simulink model "AC2DC_Converter"  (R2019a)
settings: Solver=ode23t  StartTime=0.0  StopTime=0.5  FixedStep=Ts  MaxStep=1e-4  RelTol=1e-3  EnableMultiTasking=on
PreLoadFcn:
  | pe_buck_converter_control_data;
undefined symbols (not defined in the file): RL, Ts, Tsc, Vref
libraries: fl_lib x12, nesl_utility x6, ee_lib x5, eeDcDcVoltageController x1, eePwmGenerator x1, dspstat3 x1
CloseFcn:
  | try,close(h1_pe_buck_converter_control),end
  | clear h1_pe_buck_converter_control
  | 
  | clear simlog_pe_buck_converter_control
  | clear logsout_pe_buck_converter_control
Description:
  | Buck Converter Voltage Control
  | 
  | Copyright 2017 The MathWorks, Inc.
settings Model: Creator=The MathWorks, Inc.  LastModifiedBy=jcale
settings DataIOCC: MaxDataPoints=210000  ReturnWorkspaceOutputs=off  SignalLoggingName=logsout_pe_buck_converter_control
settings OptimizationCC: LifeSpan=inf
settings DebuggingCC: UnderspecifiedInitializationDetection=Classic  MergeDetectMultiDrivingBlocksExec=none  PregeneratedLibrarySubsystemCodeDiagnostic=none  SFUnexpectedBacktrackingDiag=warning  SFNoUnconditionalDefaultTransitionDiag=warning  SFExecutionAtInitializationDiag=none  ArithmeticOperatorsInVariantConditions=warning
settings SFSimCC: SimUseLocalCustomCode=off
settings RTWCC: RTWUseLocalCustomCode=off
settings CodeAppCC: StateflowObjectComments=on
settings GRTTargetCC: TargetLangStandard=C89/C90 (ANSI)  GeneratePreprocessorConditionals=Disable all
settings ConfigComp: CovMetricSettings=dw  CovHtmlReporting=on  CovSaveCumulativeToWorkspaceVar=on  CovSaveSingleToWorkspaceVar=on  CovExternalEMLEnable=off
settings SimscapeCC: SimscapeNormalizeSystem=off  SimscapeLogType=all  SimscapeLogSimulationStatistics=on  SimscapeLogName=simlog_pe_buck_converter_control  SimscapeLogDataHistory=210000

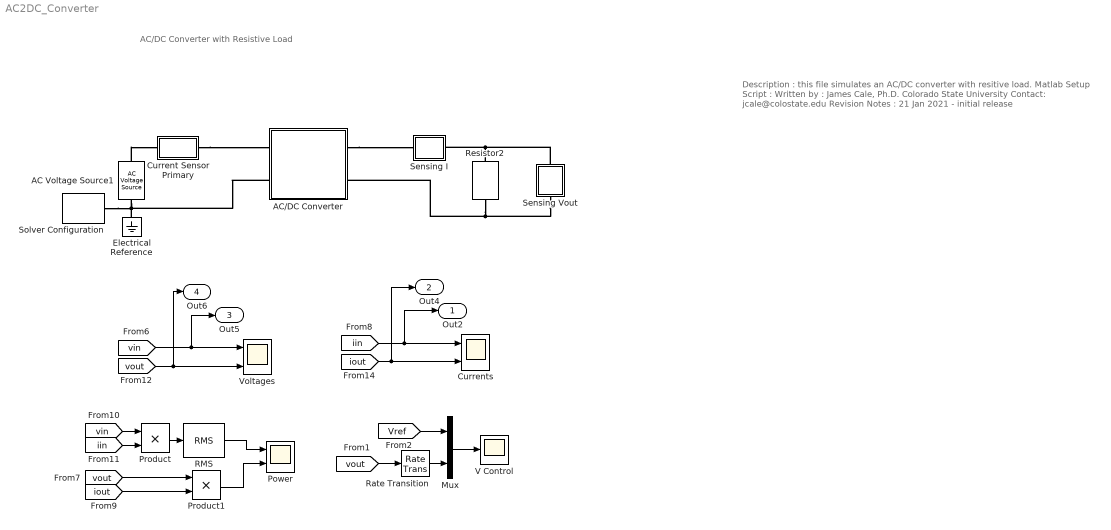
== system AC2DC_Converter ==
  note: AC/DC Converter with Resistive Load
  note: Description : this file simulates an AC/DC converter with resitive load.
      |
      | Matlab Setup Script :
      |
      | Written by :
      | James Cale, Ph.D.
      | Colorado State University
      | Contact: jcale@colostate.edu
      |
      | Revision Notes :
      | 21 Jan 2021 - initial release
  AC Voltage Source1 : fl_lib/Electrical/Electrical Sources/AC Voltage Source  amp=178 V  shift=-90 deg  frequency=60 Hz  omega=0 rad/s
  AC/DC Converter : Subsystem  mask{r_line=5e-1, l_line=1e-4, c_f=100e-6, r_f=5e-1, Kp=0.0547, Ki=8.8644}
      mask prompts: r_line "Input line resistance (Ohm)"; l_line "Input line inductance (H)"; c_f "Input filter capacitor (F)"; r_f "Input filter resistor (Ohm)"; Kp "Controller proportional gain"; Ki "Controller integrator gain"
      mask Display:
      | %disp('AC/DC Converter')
      | %pos = get_param(gcb,'Position')
      | %plot([pos(1) pos(2)],[pos(3) pos(4)])
      | plot([0.25 0.75], [.25 .25])
      | plot([0.75 0.75], [.25 0.75])
      | plot([0.75 0.25], [0.75 0.75])
      | plot([0.25 0.25], [0.75 .25])
      | plot([0.25 0.25], [0.75 .25])
      | 
      | plot([0.25 0.75], [0.25 .75])
      | 
      | text(.35,.62, '{\fontsize{20}~}','texmode','on')
      | text(.6,.45, '{\fontsize{20}-}','texmode','on')
  Current Sensor Primary : Subsystem
      mask Display: disp('v, i', 'texmode','on')
  Currents : Scope  NumInputPorts=2
  Electrical Reference : fl_lib/Electrical/Electrical Elements/Electrical Reference
  Mux : Mux  Inputs=2
  Power : Scope  NumInputPorts=2
  Product : Product
  Product1 : Product
  RMS : dspstat3/RMS  run=on  directionMode=Each column  dimension=1  InputProcessing=Columns as channels (frame based)  reset_popup=None
  Rate Transition : RateTransition  OutPortSampleTime=Tsc
  Resistor2 : fl_lib/Electrical/Electrical Elements/Resistor  R=RL Ohm  i_specify=off  i_priority=None  i=0 A  i_nominal_specify=off  i_nominal_unit=A  i_nominal_value=1  v_specify=off  v_priority=None  v=0 V  v_nominal_specify=off  v_nominal_unit=V  v_nominal_value=1
  Sensing Vout : Subsystem
      mask Display:
      | disp('v')
      | %port_label('Lconn',1,'+')
      | %port_label('Rconn',1,'-')
  Sensing I : Subsystem
      mask Display:
      | disp('i')
      | %port_label('Lconn',1,'+')
      | %port_label('Rconn',1,'-')
  Solver Configuration : nesl_utility/Solver Configuration  PhysicalDomain=network_engine_domain  SubClassName=solver  LeftPortType=input  RightPortType=generic  Tones=[]  Harmonics=[]  SimulateNoise=off  Profile=off  UseLocalSampling=off  EnableSwitchedLinearOptims=on  FrequencyDomain=off  UseCCode=off  RelTol=0.001  AbsTol=1e-06  MinStep=1e-09  ToWorkspace=off  RevertToSquareIcSolve=off  NumHomotopyIterations=100  PhasorMode=off  PhasorModeNumHarmonics=1  DoDC=off  ResidualTolerance=1e-9  UseLocalSolver=on  LocalSolverChoice=NE_BACKWARD_EULER_ADVANCER  LocalSolverSampleTime=Ts  DoFixedCost=on  MaxNonlinIter=3  MaxModeIter=2  LinearAlgebra=auto  EquationFormulation=NE_TIME_EF  DelaysMemoryBudget=1024  AutomaticFiltering=on  FilteringTimeConstant=0.001  PartitionStorageMethod=AS_NEEDED  PartitionMemoryBudget=1024  PartitionMethod=FAST
  V Control : Scope
  Voltages : Scope  NumInputPorts=2
  Out2 : Outport  SignalName=iin  InitialOutput=0
  Out4 : Outport  Port=2  SignalName=iout  InitialOutput=0
  Out5 : Outport  Port=3  SignalName=vin  InitialOutput=0
  Out6 : Outport  Port=4  SignalName=vout  InitialOutput=0
  wires:
  [vout] -> Rate Transition/1
  Mux/1 -> V Control/1
  [Vref] -> Mux/1
  Rate Transition/1 -> Mux/2
  Product/1 -> RMS/1
  [vout] -> Voltages/2, Out6/1
  [iin] -> Currents/1, Out2/1
  [iout] -> Currents/2, Out4/1
  [vin] -> Voltages/1, Out5/1
  RMS/1 -> Power/1
  [vout] -> Product1/1
  [iout] -> Product1/2
  [vin] -> Product/1
  [iin] -> Product/2
  Product1/1 -> Power/2
  connections:
  Resistor2/RConn1 -- AC/DC Converter/RConn2 -- Sensing Vout/RConn1
  Electrical Reference/LConn1 -- Solver Configuration/RConn1 -- AC/DC Converter/LConn2 -- AC Voltage Source1/RConn1
  AC Voltage Source1/LConn1 -- Current Sensor Primary/LConn1
  Current Sensor Primary/RConn1 -- AC/DC Converter/LConn1
  AC/DC Converter/RConn1 -- Sensing I/LConn1
  Sensing Vout/LConn1 -- Resistor2/LConn1 -- Sensing I/RConn1

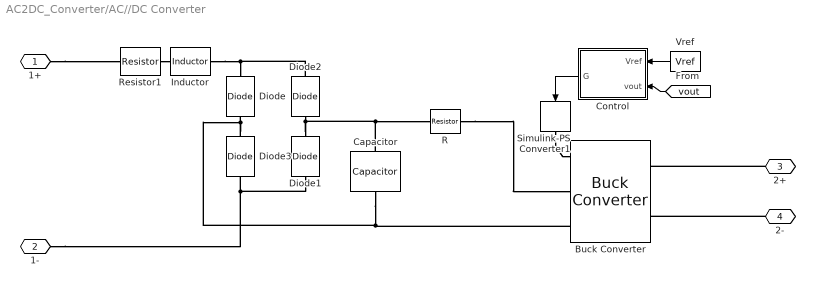
== system AC2DC_Converter/AC//DC Converter ==
  Buck Converter : ee_lib/Semiconductors & Converters/Converters/Buck Converter  device_type=3  Vf=0.8 V  Ron=0.001 Ohm  Rds=0.001 Ohm  Goff=1e-5 1/Ohm  Vth=0.5 V  Vgt=1 V  Vgt_off=-1 V  Ih=1 A  diode_param=2  diode_Vf=0.8 V  diode_Ron=0.001 Ohm  diode_Goff=1e-5 1/Ohm  diode_C=50 nF  diode_iRM=-235 A  diode_iF=300 A  diode_idot=-50 A/us  diode_trr_param=1  diode_trr_factor=3  diode_trr=15 us  diode_Qrr=1500 s*uA  Lf=3.7e-2 H  Cf=1e-5 F  Rf=0.01 Ohm  snubber_type=0  Rs=0.1 Ohm  Cs=1e-7 F
      settings: SourceProductName=Simscape Electrical  SourceProductBaseCode=PS
  Capacitor : fl_lib/Electrical/Electrical Elements/Capacitor  c=c_f F  r=1e-6 Ohm  g=0 1/Ohm  i_specify=off  i_priority=None  i=0 A  i_nominal_specify=off  i_nominal_unit=A  i_nominal_value=1  v_specify=off  v_priority=None  v=0 V  v_nominal_specify=off  v_nominal_unit=V  v_nominal_value=1  vc_specify=off  vc_priority=High  vc=0 V  vc_nominal_specify=off  vc_nominal_unit=V  vc_nominal_value=1
  Control : Subsystem
  Diode : ee_lib/Semiconductors & Converters/Diode  ModelType=ee.enum.diode.modelType.pwl  Vf=.5 V  Ron=0.2 Ohm  Goff=1e-8 S  prmExp=1  I12=[.0137, .545] A  V12=[.6, .7] V  IS=1e-12 A  ec=1  I1=0.0137 A  V1=0.6 V  RS=0.01 Ohm  Tmeas=25 degC  N_series=1  N_parallel=1  Rz=0.3 Ohm  BV=inf V  C_param=1  CJ=5 pF  CJ0=5 pF  VJ=1 V  Mgrad=0.5  Vvec=[.1, 10, 100] V  Cvec=[3.5, 1, .4] pF  FC=0.5  Q_param=ee.enum.diode.recoveryParam.off  iRM=-7.15 A  iF=4 A  didt=-750 A/us  trr_factor=3  trr=115 ns  Qrr=1500 s*uA  TT=50 ns  tau=100 ns  T_param=1  IS_T2=1.25e-7 A  I1_T2=0.245 A  V1_T2=0.5 V  Tmeas2=125 degC  EG_param=1  EG=1.11 eV  XTI_param=1  XTI=3  dBVdT=0 V/K  Tdevice=25 degC  i_specify=off  i_priority=None  i=0 A  i_nominal_specify=off  i_nominal_unit=A  i_nominal_value=1  v_specify=off  v_priority=None  v=0 V  v_nominal_specify=off  v_nominal_unit=V  v_nominal_value=1  i_capacitor_specify=off  i_capacitor_priority=High  i_capacitor=0 A  i_capacitor_nominal_specify=off  i_capacitor_nominal_unit=A  i_capacitor_nominal_value=1  v_capacitor_specify=off  v_capacitor_priority=None  v_capacitor=0 V  v_capacitor_nominal_specify=off  v_capacitor_nominal_unit=V  v_capacitor_nominal_value=1  power_dissipated_specify=off  power_dissipated_priority=None  power_dissipated=0 W  power_dissipated_nominal_specify=off  power_dissipated_nominal_unit=W  power_dissipated_nominal_value=1  Rth=[0, 10] K/W  thermal_mass_parameterization=ee.enum.thermalNetwork.timeconstant  thermal_mass=[0, 1] J/K  thermal_time_constant=[0, 10] s  thermal_mass_initial_temperatures=[25, 25] degC
      settings: SourceProductName=Simscape Electrical
  Diode1 : ee_lib/Semiconductors & Converters/Diode  ModelType=ee.enum.diode.modelType.pwl  Vf=.5 mV  Ron=0.2 Ohm  Goff=1e-8 S  prmExp=1  I12=[.0137, .545] A  V12=[.6, .7] V  IS=1e-12 A  ec=1  I1=0.0137 A  V1=0.6 V  RS=0.01 Ohm  Tmeas=25 degC  N_series=1  N_parallel=1  Rz=0.3 Ohm  BV=inf V  C_param=1  CJ=5 pF  CJ0=5 pF  VJ=1 V  Mgrad=0.5  Vvec=[.1, 10, 100] V  Cvec=[3.5, 1, .4] pF  FC=0.5  Q_param=ee.enum.diode.recoveryParam.off  iRM=-7.15 A  iF=4 A  didt=-750 A/us  trr_factor=3  trr=115 ns  Qrr=1500 s*uA  TT=50 ns  tau=100 ns  T_param=1  IS_T2=1.25e-7 A  I1_T2=0.245 A  V1_T2=0.5 V  Tmeas2=125 degC  EG_param=1  EG=1.11 eV  XTI_param=1  XTI=3  dBVdT=0 V/K  Tdevice=25 degC  i_specify=off  i_priority=None  i=0 A  i_nominal_specify=off  i_nominal_unit=A  i_nominal_value=1  v_specify=off  v_priority=None  v=0 V  v_nominal_specify=off  v_nominal_unit=V  v_nominal_value=1  i_capacitor_specify=off  i_capacitor_priority=High  i_capacitor=0 A  i_capacitor_nominal_specify=off  i_capacitor_nominal_unit=A  i_capacitor_nominal_value=1  v_capacitor_specify=off  v_capacitor_priority=None  v_capacitor=0 V  v_capacitor_nominal_specify=off  v_capacitor_nominal_unit=V  v_capacitor_nominal_value=1  power_dissipated_specify=off  power_dissipated_priority=None  power_dissipated=0 W  power_dissipated_nominal_specify=off  power_dissipated_nominal_unit=W  power_dissipated_nominal_value=1  Rth=[0, 10] K/W  thermal_mass_parameterization=ee.enum.thermalNetwork.timeconstant  thermal_mass=[0, 1] J/K  thermal_time_constant=[0, 10] s  thermal_mass_initial_temperatures=[25, 25] degC
      settings: SourceProductName=Simscape Electrical
  Diode2 : ee_lib/Semiconductors & Converters/Diode  ModelType=ee.enum.diode.modelType.pwl  Vf=.5 V  Ron=0.2 Ohm  Goff=1e-8 S  prmExp=1  I12=[.0137, .545] A  V12=[.6, .7] V  IS=1e-12 A  ec=1  I1=0.0137 A  V1=0.6 V  RS=0.01 Ohm  Tmeas=25 degC  N_series=1  N_parallel=1  Rz=0.3 Ohm  BV=inf V  C_param=1  CJ=5 pF  CJ0=5 pF  VJ=1 V  Mgrad=0.5  Vvec=[.1, 10, 100] V  Cvec=[3.5, 1, .4] pF  FC=0.5  Q_param=ee.enum.diode.recoveryParam.off  iRM=-7.15 A  iF=4 A  didt=-750 A/us  trr_factor=3  trr=115 ns  Qrr=1500 s*uA  TT=50 ns  tau=100 ns  T_param=1  IS_T2=1.25e-7 A  I1_T2=0.245 A  V1_T2=0.5 V  Tmeas2=125 degC  EG_param=1  EG=1.11 eV  XTI_param=1  XTI=3  dBVdT=0 V/K  Tdevice=25 degC  i_specify=off  i_priority=None  i=0 A  i_nominal_specify=off  i_nominal_unit=A  i_nominal_value=1  v_specify=off  v_priority=None  v=0 V  v_nominal_specify=off  v_nominal_unit=V  v_nominal_value=1  i_capacitor_specify=off  i_capacitor_priority=High  i_capacitor=0 A  i_capacitor_nominal_specify=off  i_capacitor_nominal_unit=A  i_capacitor_nominal_value=1  v_capacitor_specify=off  v_capacitor_priority=None  v_capacitor=0 V  v_capacitor_nominal_specify=off  v_capacitor_nominal_unit=V  v_capacitor_nominal_value=1  power_dissipated_specify=off  power_dissipated_priority=None  power_dissipated=0 W  power_dissipated_nominal_specify=off  power_dissipated_nominal_unit=W  power_dissipated_nominal_value=1  Rth=[0, 10] K/W  thermal_mass_parameterization=ee.enum.thermalNetwork.timeconstant  thermal_mass=[0, 1] J/K  thermal_time_constant=[0, 10] s  thermal_mass_initial_temperatures=[25, 25] degC
      settings: SourceProductName=Simscape Electrical
  Diode3 : ee_lib/Semiconductors & Converters/Diode  ModelType=ee.enum.diode.modelType.pwl  Vf=.5 V  Ron=0.2 Ohm  Goff=1e-8 S  prmExp=1  I12=[.0137, .545] A  V12=[.6, .7] V  IS=1e-12 A  ec=1  I1=0.0137 A  V1=0.6 V  RS=0.01 Ohm  Tmeas=25 degC  N_series=1  N_parallel=1  Rz=0.3 Ohm  BV=inf V  C_param=1  CJ=5 pF  CJ0=5 pF  VJ=1 V  Mgrad=0.5  Vvec=[.1, 10, 100] V  Cvec=[3.5, 1, .4] pF  FC=0.5  Q_param=ee.enum.diode.recoveryParam.off  iRM=-7.15 A  iF=4 A  didt=-750 A/us  trr_factor=3  trr=115 ns  Qrr=1500 s*uA  TT=50 ns  tau=100 ns  T_param=1  IS_T2=1.25e-7 A  I1_T2=0.245 A  V1_T2=0.5 V  Tmeas2=125 degC  EG_param=1  EG=1.11 eV  XTI_param=1  XTI=3  dBVdT=0 V/K  Tdevice=25 degC  i_specify=off  i_priority=None  i=0 A  i_nominal_specify=off  i_nominal_unit=A  i_nominal_value=1  v_specify=off  v_priority=None  v=0 V  v_nominal_specify=off  v_nominal_unit=V  v_nominal_value=1  i_capacitor_specify=off  i_capacitor_priority=High  i_capacitor=0 A  i_capacitor_nominal_specify=off  i_capacitor_nominal_unit=A  i_capacitor_nominal_value=1  v_capacitor_specify=off  v_capacitor_priority=None  v_capacitor=0 V  v_capacitor_nominal_specify=off  v_capacitor_nominal_unit=V  v_capacitor_nominal_value=1  power_dissipated_specify=off  power_dissipated_priority=None  power_dissipated=0 W  power_dissipated_nominal_specify=off  power_dissipated_nominal_unit=W  power_dissipated_nominal_value=1  Rth=[0, 10] K/W  thermal_mass_parameterization=ee.enum.thermalNetwork.timeconstant  thermal_mass=[0, 1] J/K  thermal_time_constant=[0, 10] s  thermal_mass_initial_temperatures=[25, 25] degC
      settings: SourceProductName=Simscape Electrical
  Inductor : fl_lib/Electrical/Electrical Elements/Inductor  l=l_line H  r=0 Ohm  g=1e-9 1/Ohm  i_specify=off  i_priority=None  i=0 A  i_nominal_specify=off  i_nominal_unit=A  i_nominal_value=1  v_specify=off  v_priority=None  v=0 V  v_nominal_specify=off  v_nominal_unit=V  v_nominal_value=1  i_L_specify=off  i_L_priority=High  i_L=0 A  i_L_nominal_specify=off  i_L_nominal_unit=A  i_L_nominal_value=1
  R : fl_lib/Electrical/Electrical Elements/Resistor  R=r_f Ohm  i_specify=off  i_priority=None  i=0 A  i_nominal_specify=off  i_nominal_unit=A  i_nominal_value=1  v_specify=off  v_priority=None  v=0 V  v_nominal_specify=off  v_nominal_unit=V  v_nominal_value=1
      settings: SourceProductName=Foundation Library
  Resistor1 : fl_lib/Electrical/Electrical Elements/Resistor  R=r_line Ohm  i_specify=off  i_priority=None  i=0 A  i_nominal_specify=off  i_nominal_unit=A  i_nominal_value=1  v_specify=off  v_priority=None  v=0 V  v_nominal_specify=off  v_nominal_unit=V  v_nominal_value=1
  Simulink-PS Converter1 : nesl_utility/Simulink-PS Converter  PhysicalDomain=network_engine_domain  SubClassName=ps_input  LeftPortType=input  RightPortType=output  PseudoPeriodic=off  Frequencies=[]  NoiseDistribution=none  NoiseParameters=[]  Unit=1  AffineConversion=off  FilteringAndDerivatives=provide  SimscapeFilterOrder=1  InputFilterTimeConstant=0.001  UdotUserProvided=0
  Vref : Constant  Value=Vref  SampleTime=Ts
  1+ : PMIOPort  Side=Left
  1- : PMIOPort  Port=2  Side=Left
  2+ : PMIOPort  Port=3  Side=Right
  2- : PMIOPort  Port=4  Side=Right
  wires:
  [vout] -> Control/2(vout)
  Control/1(G) -> Simulink-PS Converter1/1
  Vref/1 -> Control/1(Vref)
  connections:
  2-/RConn1 -- Buck Converter/RConn2
  1+/RConn1 -- Resistor1/LConn1
  2+/RConn1 -- Buck Converter/RConn1
  Simulink-PS Converter1/RConn1 -- Buck Converter/LConn1
  Diode3/RConn1 -- 1-/RConn1 -- Diode1/LConn1
  Resistor1/RConn1 -- Inductor/LConn1
  R/RConn1 -- Buck Converter/LConn2
  Diode/RConn1 -- Diode2/LConn1 -- Inductor/RConn1
  Diode/LConn1 -- Capacitor/RConn1 -- Buck Converter/LConn3 -- Diode3/LConn1
  Capacitor/LConn1 -- Diode2/RConn1 -- Diode1/RConn1 -- R/LConn1

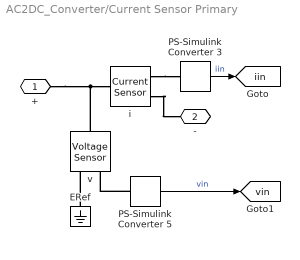
== system AC2DC_Converter/Current Sensor Primary ==
  ERef : fl_lib/Electrical/Electrical Elements/Electrical Reference
  PS-Simulink Converter 3 : nesl_utility/PS-Simulink Converter  PhysicalDomain=network_engine_domain  SubClassName=ps_output  LeftPortType=input  RightPortType=output  PseudoPeriodic=off  Frequencies=[]  Unit=1  AffineConversion=off
  PS-Simulink Converter 5 : nesl_utility/PS-Simulink Converter  PhysicalDomain=network_engine_domain  SubClassName=ps_output  LeftPortType=input  RightPortType=output  PseudoPeriodic=off  Frequencies=[]  Unit=1  AffineConversion=off
  i : fl_lib/Electrical/Electrical Sensors/Current Sensor
  v : fl_lib/Electrical/Electrical Sensors/Voltage Sensor
  + : PMIOPort  Side=Left
  - : PMIOPort  Port=2  Side=Right
  tag scope: iin=global, vin=global
  wires:
  PS-Simulink Converter 3/1 -> [iin]  "iin"
  PS-Simulink Converter 5/1 -> [vin]  "vin"
  connections:
  i/RConn2 -- -/RConn1
  +/RConn1 -- v/LConn1 -- i/LConn1
  i/RConn1 -- PS-Simulink Converter 3/LConn1
  PS-Simulink Converter 5/LConn1 -- v/RConn1
  ERef/LConn1 -- v/RConn2

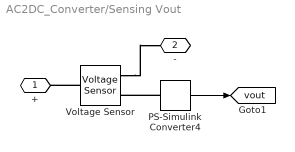
== system AC2DC_Converter/Sensing Vout ==
  PS-Simulink Converter4 : nesl_utility/PS-Simulink Converter  PhysicalDomain=network_engine_domain  SubClassName=ps_output  LeftPortType=input  RightPortType=output  PseudoPeriodic=off  Frequencies=[]  Unit=V  AffineConversion=off
  Voltage Sensor : fl_lib/Electrical/Electrical Sensors/Voltage Sensor
      settings: SourceProductName=Foundation Library
  + : PMIOPort  Side=Left
  - : PMIOPort  Port=2  Side=Right
  tag scope: vout=global
  wires:
  PS-Simulink Converter4/1 -> [vout]
  connections:
  Voltage Sensor/LConn1 -- +/RConn1
  Voltage Sensor/RConn2 -- -/RConn1
  PS-Simulink Converter4/LConn1 -- Voltage Sensor/RConn1

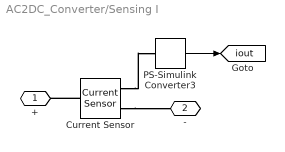
== system AC2DC_Converter/Sensing I ==
  Current Sensor : fl_lib/Electrical/Electrical Sensors/Current Sensor
  PS-Simulink Converter3 : nesl_utility/PS-Simulink Converter  PhysicalDomain=network_engine_domain  SubClassName=ps_output  LeftPortType=input  RightPortType=output  PseudoPeriodic=off  Frequencies=[]  Unit=A  AffineConversion=off
  + : PMIOPort  Side=Left
  - : PMIOPort  Port=2  Side=Right
  tag scope: iout=global
  wires:
  PS-Simulink Converter3/1 -> [iout]
  connections:
  Current Sensor/RConn2 -- -/RConn1
  Current Sensor/LConn1 -- +/RConn1
  Current Sensor/RConn1 -- PS-Simulink Converter3/LConn1

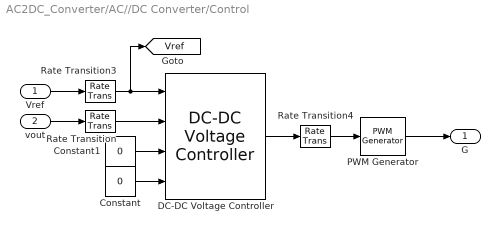
== system AC2DC_Converter/AC//DC Converter/Control ==
  Vref : Inport
  vout : Inport  Port=2
  Constant : Constant  Value=0
  Constant1 : Constant  Value=0
  DC-DC Voltage Controller : eeDcDcVoltageController/DC-DC Voltage Controller  Kp=Kp  Ki=Ki  Kaw=1  up=0.95  lo=0  Ts=Tsc  Tf=0.001  ActVdcFilter=off
      settings: SourceProductName=Simscape Electrical  SourceProductBaseCode=PS
  PWM Generator : eePwmGenerator/PWM Generator  CarrCount=Up  Tper=1e-4  Ts=Ts
      settings: SourceProductName=Simscape Electrical
  Rate Transition : RateTransition  OutPortSampleTime=Tsc
  Rate Transition3 : RateTransition  OutPortSampleTime=Tsc
  Rate Transition4 : RateTransition  OutPortSampleTime=Ts
  G : Outport
  tag scope: Vref=global
  wires:
  Vref/1 -> Rate Transition3/1
  Rate Transition3/1 -> [Vref], DC-DC Voltage Controller/1
  vout/1 -> Rate Transition/1
  PWM Generator/1 -> G/1
  DC-DC Voltage Controller/1 -> Rate Transition4/1
  Rate Transition4/1 -> PWM Generator/1
  Constant1/1 -> DC-DC Voltage Controller/3
  Constant/1 -> DC-DC Voltage Controller/4
  Rate Transition/1 -> DC-DC Voltage Controller/2
